simulink model "MPC_accessible_state"  (R2022a)
settings: Solver=VariableStepAuto  StartTime=0.0  StopTime=10.0  RelTol=1e-3
values from neighbouring files (symbols this model uses):
  condDiscMat = BuildCondendsedMPCmatrices(discreteMat,r_Kalman,q_Kalman,F,f,PH)    [MAIN_MIMO.m]    (also in backupMain.m = BuildCondendsedMPCmatrices(discreteMat,r,q,F,f,PH); test.m = BuildCondendsedMPCmatrices(discreteMat,r,q,F,f,PH))
  discreteModel = c2d(continuousModel, info.Ts)    [MAIN_MIMO.m]    (also in backupMain.m; nonLinearPatient_main.m; test.m)
  PH = 200    [MAIN_MIMO.m]    (also in backupMain.m; nonLinearPatient_main.m; test.m)
undefined symbols (not defined in the file or in its folder): info, myMPC_dist, op
settings Model: Creator=user  LastModifiedBy=user

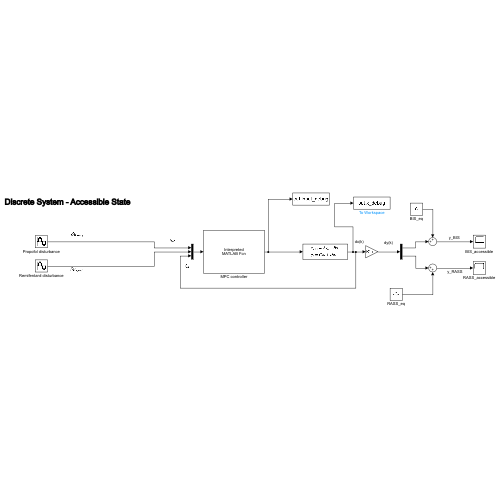
[thumbnail: Simulink's stored preview of the top-level diagram]
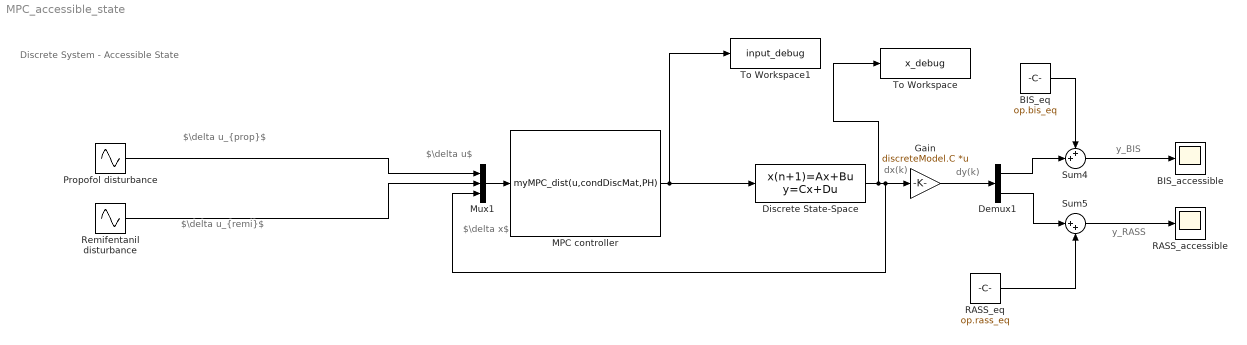
== system MPC_accessible_state ==
  note: $\delta u$
  note: $\delta x$
  note: y_RASS
  note: y_BIS
  note: dx(k)
  note: Discrete System - Accessible State
  note: dy(k)
  note: $\delta u_{remi}$
  note: $\delta u_{prop}$
  BIS_accessible : Scope
  BIS_eq : Constant  Value=op.bis_eq
  Demux1 : Demux  Outputs=2
  Discrete State-Space : DiscreteStateSpace  A=discreteModel.A  B=discreteModel.B  C=eye(size(discreteModel.A))  D=zeros(size(discreteModel.A,1),size(discreteModel.B,2))  SampleTime=info.Ts
  Gain : Gain  Gain=discreteModel.C  Multiplication=Matrix(K*u)
  MPC controller : MATLABFcn  MATLABFcn=myMPC_dist(u,condDiscMat,PH)  OutputDimensions=2
  Mux1 : Mux  Inputs=3
  Propofol disturbance : Sin  Amplitude=0.3*op.propofol_eq  Frequency=1/500  SampleTime=info.Ts
  RASS_accessible : Scope
  RASS_eq : Constant  Value=op.rass_eq
  Remifentanil disturbance : Sin  Amplitude=0.3*op.remifentanil_eq  Frequency=1/700  SampleTime=info.Ts
  Sum4 : Sum  Inputs=++|
  Sum5 : Sum  Inputs=|++
  To Workspace : ToWorkspace  VariableName=x_debug  SaveFormat=Structure With Time  SampleTime=-1
  To Workspace1 : ToWorkspace  VariableName=input_debug  SaveFormat=Structure With Time  SampleTime=-1
  wires:
  Sum4/1 -> BIS_accessible/1
  BIS_eq/1 -> Sum4/1
  Demux1/1 -> Sum4/2
  Mux1/1 -> MPC controller/1
  Sum5/1 -> RASS_accessible/1
  Gain/1 -> Demux1/1
  RASS_eq/1 -> Sum5/2
  Remifentanil disturbance/1 -> Mux1/2
  Demux1/2 -> Sum5/1
  Propofol disturbance/1 -> Mux1/1
  MPC controller/1 -> Discrete State-Space/1, To Workspace1/1
  Discrete State-Space/1 -> To Workspace/1, Mux1/3, Gain/1
